simulink model "CK_index_center_main"  (R2023a)
settings: Solver=VariableStepAuto  StartTime=0.0  StopTime=100  RelTol=1e-3
undefined symbols (not defined in the file): a0, a1, a2, a_i_notTop, a_i_Top, Alpha, Alpha1, Alpha2, Alpha3, b0, b1, b2, Cr, d1, d2, DCLV3, DCLV3signal, DCyt, ds, DSstemcells, dw, K1, K2, Kh1, Kh2, n, ra, rclv, rclvs, rcyt, receptor_i1, receptor_i2, receptor_i3, receptor_i4, receptor_i5, receptor_i6, receptor_i7, receptor_i8, rsc, rw, V1, Vh1
settings Model: Creator=mosuk  LastModifiedBy=mosuk

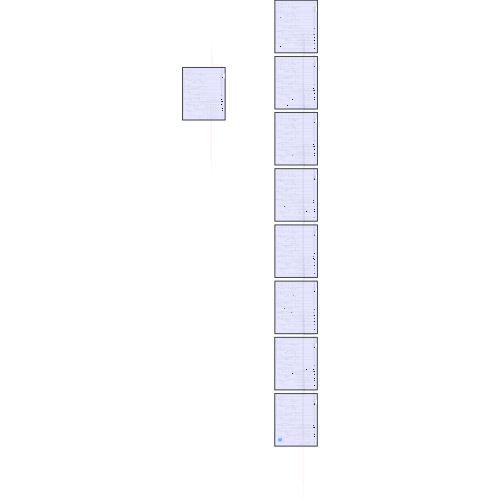
[thumbnail: Simulink's stored preview of the top-level diagram]
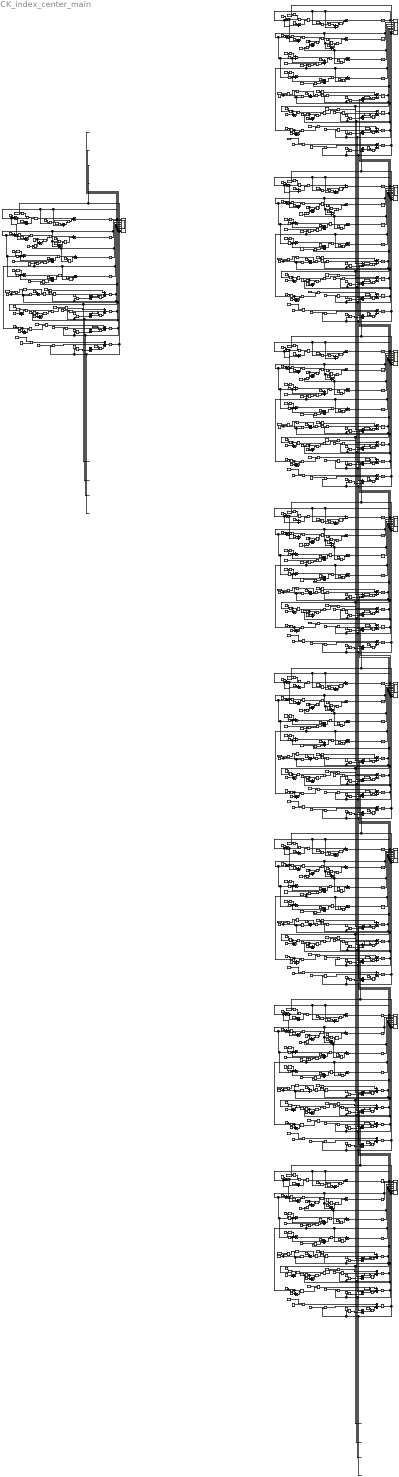
== system CK_index_center_main ==
  note: a_i_notTop
  note: i = 2
  note: i = 3
  note: i = 1
  note: i = 1
  note: i = 4
  note: i = 5
  note: i = 6
  note: i = 7
  note: i = 8
  Constant{100,148,244,292,340,388,436,484,532} (9 alike) : Constant  Value=a1
  Constant{101,149,245,293,341,389,437,485,533} (9 alike) : Constant  Value=ra
  Constant{102,150,246,294,342,390,438,486,534} (9 alike) : Constant  Value=a2
  Constant{103,151,247,295,343,391,439,487,535} (9 alike) : Constant  Value=b1
  Constant{104,152,248,296,344,392,440,488,536} (9 alike) : Constant  Value=n
  Constant{105,109,116,123,125,127,136,153,157,164,171,173,175,184,249,253,260,267,269,271,280,297,301,308,315,317,319,322,324..326,328,345,349,356,363,365,367,376,393,397,404,411,413,415,424,441,445,452,459,461,463,472,489,493,500,507,509,511,520,537,541,548,555,557,559,568} (67 alike) : Constant
  Constant{106,154,250,298,346,394,442,490,538} (9 alike) : Constant  Value=b2
  Constant{107,155,251,299,347,395,443,491,539} (9 alike) : Constant  Value=b0
  Constant{99,108,147,156,243,252,291,300,339,348,387,396,435,444,483,492,531,540} (18 alike) : Constant  Value=10
  Constant{110,158,254,302,350,398,446,494,542} (9 alike) : Constant  Value=d2
  Constant{111,159,255,303,351,399,447,495,543} (9 alike) : Constant  Value=ds
  Constant{112,160,256,304,352,400,448,496,544} (9 alike) : Constant  Value=Alpha1
  Constant{113,161,257,305,353,401,449,497,545} (9 alike) : Constant  Value=rw
  Constant{114,162,258,306,354,402,450,498,546} (9 alike) : Constant  Value=Alpha3
  Constant{115,163,259,307,355,403,451,499,547} (9 alike) : Constant  Value=Cr
  Constant{117,131,165,179,357,371,405,419,453,467,501,515,549,563} (14 alike) : Constant  Value=a_i_notTop
  Constant{118,166,262,310,358,406,454,502,550} (9 alike) : Constant  Value=rclvs
  Constant{119,167,263,311,359,407,455,503,551} (9 alike) : Constant  Value=Kh1
  Constant{120,168,264,312,360,408,456,504,552} (9 alike) : Constant  Value=d1
  Constant{121,169,265,313,361,409,457,505,553} (9 alike) : Constant  Value=Alpha2
  Constant{122,170,266,314,362,410,458,506,554} (9 alike) : Constant  Value=rclv
  Constant{124,172,268,316,364,412,460,508,556} (9 alike) : Constant  Value=rsc
  Constant{126,174,270,318,366,414,462,510,558} (9 alike) : Constant  Value=rcyt
  Constant{128,176,272,320,368,416,464,512,560} (9 alike) : Constant  Value=dw
  Constant{129,177,273,321,369,417,465,513,561} (9 alike) : Constant  Value=Kh2
  Constant{130,132..134,178,180..182,274,276..278,370,372..374,418,420..422,466,468..470,514,516..518,562,564..566} (32 alike) : Constant  Value=2
  Constant{135,183,279,327,375,423,471,519,567} (9 alike) : Constant  Value=Vh1
  Constant{137,185,281,329,377,425,473,521,569} (9 alike) : Constant  Value=DCLV3
  Constant{138,186,282,330,378,426,474,522,570} (9 alike) : Constant  Value=a0
  Constant{139,187,283,331,379,427,475,523,571} (9 alike) : Constant  Value=Alpha
  Constant{140,188,284,332,380,428,476,524,572} (9 alike) : Constant  Value=DCLV3signal
  Constant{141,189,285,333,381,429,477,525,573} (9 alike) : Constant  Value=DCyt
  Constant{142,190,286,334,382,430,478,526,574} (9 alike) : Constant  Value=DSstemcells
  Constant{143,191,287,335,383,431,479,527,575} (9 alike) : Constant  Value=V1
  Constant144 : Constant  Value=receptor_i3
  Constant{97,145,241,289,337,385,433,481,529} (9 alike) : Constant  Value=K1
  Constant{98,146,242,290,338,386,434,482,530} (9 alike) : Constant  Value=K2
  Constant240 : Constant  Value=receptor_i1
  Constant{261,275,309,323} (4 alike) : Constant  Value=a_i_Top
  Constant288 : Constant  Value=receptor_i1
  Constant336 : Constant  Value=receptor_i4
  Constant384 : Constant  Value=receptor_i5
  Constant432 : Constant  Value=receptor_i6
  Constant480 : Constant  Value=receptor_i7
  Constant528 : Constant  Value=receptor_i8
  Constant96 : Constant  Value=receptor_i2
  Divide{22..43,55..131} (99 alike) : Product  Inputs=*/
  Integrator{16..31,40..95} (72 alike) : Integrator
  Math Function{2..3,5..11} (9 alike) : Math  Operator=pow
  Product{72..143,180..431} (324 alike) : Product
  Subtract{68,73..74,76,95,100..101,103,149,154..155,157,176,181..182,184,203,208..209,211,230,235..236,238,257,262..263,265,284,289..290,292,311,316..317,319} (36 alike) : Sum  Inputs=+-+
  Subtract{54,58,65,72,75,80..81,85,92,99,102,107,135,139,146,153,156,161..162,166,173,180,183,188..189,193,200,207,210,215..216,220,227,234,237,242..243,247,254,261,264,269..270,274,281,288,291,296..297,301,308,315,318,323} (54 alike) : Sum  Inputs=+-
  Subtract{55..56,59,61,63..64,67,71,77..79,82..83,86,88,90..91,94,98,104..106,136..137,140,142,144..145,148,152,158..160,163..164,167,169,171..172,175,179,185..187,190..191,194,196,198..199,202,206,212..214,217..218,221,223,225..226,229,233,239..241,244..245,248,250,252..253,256,260,266..268,271..272,275,277,279..280,283,287,293..295,298..299,302,304,306..307,310,314,320..322} (99 alike) : Sum
  Subtract{57,60,84,87,138,141,165,168,192,195,219,222,246,249,273,276,300,303} (18 alike) : Sum  Inputs=+++
  Subtract{62,66,69..70,89,93,96..97,143,147,150..151,170,174,177..178,197,201,204..205,224,228,231..232,251,255,258..259,278,282,285..286,305,309,312..313} (36 alike) : Sum  Inputs=++-
  i -6 : Scope  NumInputPorts=8
  i = {1..8} (8 alike) : Scope  NumInputPorts=8
  wires:
  Constant132/1 -> Product95/1
  Subtract72/1 -> Integrator23/1  "Bp'"
  Constant107/1 -> Subtract59/1
  Constant111/1 -> Product76/2, Product79/1
  Constant139/1 -> Product94/2
  Constant127/1 -> Subtract67/1
  Subtract55/1 -> Divide22/2
  Constant143/1 -> Product99/1
  Subtract76/1 -> Integrator20/1  "Sstemcells'"
  Constant130/1 -> Product93/1
  Constant116/1 -> Subtract61/1
  Product95/1 -> Subtract66/3
  Product87/1 -> Subtract76/2
  Constant133/1 -> Product96/1
  Constant138/1 -> Subtract56/1
  Divide29/1 -> Subtract58/1
  Subtract80/1 -> Integrator16/1  "A'"
  Subtract67/1 -> Divide24/2
  Math Function2/1 -> Product105/2
  Constant122/1 -> Product81/1
  Divide31/1 -> Product85/1
  Product100/1 -> Subtract74/3
  Divide24/1 -> Product89/2
  Constant102/1 -> Product105/1
  Constant120/1 -> Product83/1
  Divide23/1 -> Subtract65/2
  Subtract69/1 -> Product102/2
  Product89/1 -> Subtract76/1
  Divide32/1 -> Product85/2
  Product86/1 -> Subtract64/2, Divide32/1
  Subtract75/1 -> Subtract77/2, Product84/2  "B"
  Subtract70/1 -> Product103/2
  Constant137/1 -> Product101/1
  Product81/1 -> Subtract73/2
  Subtract74/1 -> Integrator18/1  "CLV3signal'"
  Constant118/1 -> Product80/1
  Constant136/1 -> Subtract78/1, Divide26/1
  Constant106/1 -> Product74/1
  Divide22/1 -> Subtract65/1
  Constant98/1 -> Subtract79/1
  Constant114/1 -> Product89/1
  Product73/1 -> Divide23/1
  Constant117/1 -> Product76/1
  Integrator20/1 -> Product86/2, Product79/2, Product78/2, Subtract177/2, i = 2/7, Subtract96/1, Product96/2, Product87/2  "2Sstemcells"
  Product107/1 -> Subtract60/2, Subtract59/2
  Product74/1 -> Subtract60/3
  Product76/1 -> Product78/1
  Product82/1 -> Subtract73/1
  Integrator16/1 -> Product106/2, Product94/1, i = 2/3  "2A"
  Product77/1 -> Subtract74/1
  Divide28/1 -> Subtract80/1
  Constant109/1 -> Subtract60/1
  Subtract79/1 -> Divide27/2
  Constant126/1 -> Product91/1
  Subtract62/1 -> Product101/2
  Product99/1 -> Divide27/1
  Subtract57/1 -> Divide28/2
  Constant115/1 -> Product90/2
  Constant108/1 -> Subtract54/1
  Divide30/1 -> Product77/2
  Integrator21/1 -> Product92/1, Subtract178/2, i = 2/8, Subtract97/1, Product97/2, Product91/2  "2Cyt"
  Constant124/1 -> Product87/1
  Integrator19/1 -> Subtract89/1, Product81/2, Product93/2, Product74/2, Subtract170/2, i = 2/6  "2CLV3"
  Constant101/1 -> Product106/1
  Divide26/1 -> Product98/2
  Subtract61/1 -> Divide30/2
  Constant112/1 -> Product77/1
  Product105/1 -> Subtract57/3
  Product96/1 -> Subtract69/3
  Subtract77/1 -> Divide25/2
  Constant100/1 -> Product104/1
  Constant104/1 -> Math Function2/2
  Integrator18/1 -> Product95/2, Product80/2, Subtract93/1, Product83/2, Subtract174/2, i = 2/5  "2CLV3signal"
  Subtract78/1 -> Divide26/2
  Subtract65/1 -> Integrator22/1  "AHPTp'"
  Subtract71/1 -> Divide23/2
  Product72/1 -> Divide22/1
  Integrator22/1 -> Subtract71/2, Product73/2, Product84/1, Subtract54/2, i = 2/1  "2AHPTp"
  Product79/1 -> Subtract61/2
  Constant119/1 -> Subtract55/1
  Constant110/1 -> Product86/1
  Constant103/1 -> Product107/1
  Subtract56/1 -> Divide28/1
  Subtract64/1 -> Divide32/2
  Integrator23/1 -> Subtract79/2, Product99/2, Subtract75/2, Product107/2, Product104/2, i = 2/2  "2Bp"
  Product90/1 -> Subtract68/1
  Subtract66/1 -> Product100/2
  Subtract58/1 -> Integrator17/1  "WUS'"
  Product91/1 -> Subtract68/2
  Integrator17/1 -> Product75/2, Product88/2, Math Function2/1, i = 2/4  "2WUS"
  Constant105/1 -> Subtract57/1
  Product106/1 -> Subtract80/2
  Constant121/1 -> Product82/1
  Product85/1 -> Product82/2
  Constant125/1 -> Subtract63/1
  Product94/1 -> Subtract78/2
  Product93/1 -> Subtract62/3
  Product83/1 -> Divide31/1, Subtract63/2
  Product101/1 -> Subtract73/3
  Constant134/1 -> Product97/1
  Divide25/1 -> Product98/1
  Product97/1 -> Subtract70/3
  Constant99/1 -> Subtract75/1
  Subtract63/1 -> Divide31/2
  Product75/1 -> Subtract58/2
  Constant128/1 -> Product88/1
  Constant123/1 -> Subtract64/1
  Constant96/1 -> Product92/2
  Product78/1 -> Divide30/1
  Product84/1 -> Divide25/1
  Product104/1 -> Subtract57/2, Subtract56/2
  Constant113/1 -> Product75/1
  Product92/1 -> Product72/1
  Constant129/1 -> Subtract71/1
  Constant131/1 -> Product90/1
  Divide27/1 -> Subtract72/2
  Constant97/1 -> Subtract77/1
  Subtract73/1 -> Integrator19/1  "CLV3'"
  Constant140/1 -> Product100/1
  Subtract59/1 -> Divide29/1
  Subtract60/1 -> Divide29/2
  Constant135/1 -> Product73/1
  Constant142/1 -> Product102/1
  Product103/1 -> Subtract68/3
  Subtract68/1 -> Integrator21/1  "Cyt'"
  Constant141/1 -> Product103/1
  Subtract54/1 -> Subtract55/2, Product72/2  "AHPT"
  Product102/1 -> Subtract76/3
  Product88/1 -> Subtract67/2, Divide24/1
  Product98/1 -> Subtract72/1
  Product80/1 -> Subtract74/2
  Constant180/1 -> Product131/1
  Subtract99/1 -> Integrator31/1  "Bp'"
  Constant155/1 -> Subtract86/1
  Constant159/1 -> Product112/2, Product115/1
  Constant187/1 -> Product130/2
  Constant175/1 -> Subtract94/1
  Subtract82/1 -> Divide33/2
  Constant191/1 -> Product135/1
  Subtract103/1 -> Integrator28/1  "Sstemcells'"
  Constant178/1 -> Product129/1
  Constant164/1 -> Subtract88/1
  Product131/1 -> Subtract93/3
  Product123/1 -> Subtract103/2
  Constant181/1 -> Product132/1
  Constant186/1 -> Subtract83/1
  Divide40/1 -> Subtract85/1
  Subtract107/1 -> Integrator24/1  "A'"
  Subtract94/1 -> Divide35/2
  Math Function3/1 -> Product141/2
  Constant170/1 -> Product117/1
  Divide42/1 -> Product121/1
  Product136/1 -> Subtract101/3
  Divide35/1 -> Product125/2
  Constant150/1 -> Product141/1
  Constant168/1 -> Product119/1
  Divide34/1 -> Subtract92/2
  Subtract96/1 -> Product138/2
  Product125/1 -> Subtract103/1
  Divide43/1 -> Product121/2
  Product122/1 -> Subtract91/2, Divide43/1
  Subtract102/1 -> Subtract104/2, Product120/2  "B"
  Subtract97/1 -> Product139/2
  Constant185/1 -> Product137/1
  Product117/1 -> Subtract100/2
  Subtract101/1 -> Integrator26/1  "CLV3signal'"
  Constant166/1 -> Product116/1
  Constant184/1 -> Subtract105/1, Divide37/1
  Constant154/1 -> Product110/1
  Divide33/1 -> Subtract92/1
  Constant146/1 -> Subtract106/1
  Constant162/1 -> Product125/1
  Product109/1 -> Divide34/1
  Constant165/1 -> Product112/1
  Integrator28/1 -> Product122/2, Product115/2, Product114/2, Subtract69/2, i = 3/7, Subtract204/1, Product132/2, Product123/2  "3Sstemcells"
  Product143/1 -> Subtract87/2, Subtract86/2
  Product110/1 -> Subtract87/3
  Product112/1 -> Product114/1
  Product118/1 -> Subtract100/1
  Integrator24/1 -> Product142/2, Product130/1, i = 3/3  "3A"
  Product113/1 -> Subtract101/1
  Divide39/1 -> Subtract107/1
  Constant157/1 -> Subtract87/1
  Subtract106/1 -> Divide38/2
  Constant174/1 -> Product127/1
  Subtract89/1 -> Product137/2
  Product135/1 -> Divide38/1
  Subtract84/1 -> Divide39/2
  Constant163/1 -> Product126/2
  Constant156/1 -> Subtract81/1
  Divide41/1 -> Product113/2
  Integrator29/1 -> Subtract70/2, Product128/1, i = 3/8, Subtract205/1, Product133/2, Product127/2  "3Cyt"
  Constant172/1 -> Product123/1
  Integrator27/1 -> Subtract197/1, Product117/2, Product129/2, Product110/2, Subtract62/2, i = 3/6  "3CLV3"
  Constant149/1 -> Product142/1
  Divide37/1 -> Product134/2
  Subtract88/1 -> Divide41/2
  Constant160/1 -> Product113/1
  Product141/1 -> Subtract84/3
  Product132/1 -> Subtract96/3
  Subtract104/1 -> Divide36/2
  Constant148/1 -> Product140/1
  Constant152/1 -> Math Function3/2
  Integrator26/1 -> Product131/2, Product116/2, Subtract201/1, Product119/2, Subtract66/2, i = 3/5  "3CLV3signal"
  Subtract105/1 -> Divide37/2
  Subtract92/1 -> Integrator30/1  "AHPTp'"
  Subtract98/1 -> Divide34/2
  Product108/1 -> Divide33/1
  Integrator30/1 -> Subtract98/2, Product109/2, Product120/1, Subtract81/2, i = 3/1  "3AHPTp"
  Product115/1 -> Subtract88/2
  Constant167/1 -> Subtract82/1
  Constant158/1 -> Product122/1
  Constant151/1 -> Product143/1
  Subtract83/1 -> Divide39/1
  Subtract91/1 -> Divide43/2
  Integrator31/1 -> Subtract106/2, Product135/2, Subtract102/2, Product143/2, Product140/2, i = 3/2  "3Bp"
  Product126/1 -> Subtract95/1
  Subtract93/1 -> Product136/2
  Subtract85/1 -> Integrator25/1  "WUS'"
  Product127/1 -> Subtract95/2
  Integrator25/1 -> Product111/2, Product124/2, Math Function3/1, i = 3/4  "3WUS"
  Constant153/1 -> Subtract84/1
  Product142/1 -> Subtract107/2
  Constant169/1 -> Product118/1
  Product121/1 -> Product118/2
  Constant173/1 -> Subtract90/1
  Product130/1 -> Subtract105/2
  Product129/1 -> Subtract89/3
  Product119/1 -> Divide42/1, Subtract90/2
  Product137/1 -> Subtract100/3
  Constant182/1 -> Product133/1
  Divide36/1 -> Product134/1
  Product133/1 -> Subtract97/3
  Constant147/1 -> Subtract102/1
  Subtract90/1 -> Divide42/2
  Product111/1 -> Subtract85/2
  Constant176/1 -> Product124/1
  Constant171/1 -> Subtract91/1
  Constant144/1 -> Product128/2
  Product114/1 -> Divide41/1
  Product120/1 -> Divide36/1
  Product140/1 -> Subtract84/2, Subtract83/2
  Constant161/1 -> Product111/1
  Product128/1 -> Product108/1
  Constant177/1 -> Subtract98/1
  Constant179/1 -> Product126/1
  Divide38/1 -> Subtract99/2
  Constant145/1 -> Subtract104/1
  Subtract100/1 -> Integrator27/1  "CLV3'"
  Constant188/1 -> Product136/1
  Subtract86/1 -> Divide40/1
  Subtract87/1 -> Divide40/2
  Constant183/1 -> Product109/1
  Constant190/1 -> Product138/1
  Product139/1 -> Subtract95/3
  Subtract95/1 -> Integrator29/1  "Cyt'"
  Constant189/1 -> Product139/1
  Subtract81/1 -> Subtract82/2, Product108/2  "AHPT"
  Product138/1 -> Subtract103/3
  Product124/1 -> Subtract94/2, Divide35/1
  Product134/1 -> Subtract99/1
  Product116/1 -> Subtract101/2
  Constant276/1 -> Product203/1
  Subtract153/1 -> Integrator47/1  "Bp'"
  Constant251/1 -> Subtract140/1
  Constant255/1 -> Product184/2, Product187/1
  Constant283/1 -> Product202/2
  Constant271/1 -> Subtract148/1
  Subtract136/1 -> Divide55/2
  Constant287/1 -> Product207/1
  Subtract157/1 -> Integrator44/1  "Sstemcells'"
  Constant274/1 -> Product201/1
  Constant260/1 -> Subtract142/1
  Product203/1 -> Subtract147/3
  Product195/1 -> Subtract157/2
  Constant277/1 -> Product204/1
  Constant282/1 -> Subtract137/1
  Divide62/1 -> Subtract139/1
  Subtract161/1 -> Integrator40/1  "A'"
  Subtract148/1 -> Divide57/2
  Math Function5/1 -> Product213/2
  Constant266/1 -> Product189/1
  Divide64/1 -> Product193/1
  Product208/1 -> Subtract155/3
  Divide57/1 -> Product197/2
  Constant246/1 -> Product213/1
  Constant264/1 -> Product191/1
  Divide56/1 -> Subtract146/2
  Subtract150/1 -> Product210/2
  Product197/1 -> Subtract157/1
  Divide65/1 -> Product193/2
  Product194/1 -> Subtract145/2, Divide65/1
  Subtract156/1 -> Subtract158/2, Product192/2  "B"
  Subtract151/1 -> Product211/2
  Constant281/1 -> Product209/1
  Product189/1 -> Subtract154/2
  Subtract155/1 -> Integrator42/1  "CLV3signal'"
  Constant262/1 -> Product188/1
  Constant280/1 -> Subtract159/1, Divide59/1
  Constant250/1 -> Product182/1
  Divide55/1 -> Subtract146/1
  Constant242/1 -> Subtract160/1
  Constant258/1 -> Product197/1
  Product181/1 -> Divide56/1
  Constant261/1 -> Product184/1
  Integrator44/1 -> Product194/2, Product187/2, Product186/2, i -6/7, Product204/2, Product195/2  "0Sstemcells"
  Product215/1 -> Subtract141/2, Subtract140/2
  Product182/1 -> Subtract141/3
  Product184/1 -> Product186/1
  Product190/1 -> Subtract154/1
  Integrator40/1 -> Product214/2, Product202/1, i -6/3  "2A"
  Product185/1 -> Subtract155/1
  Divide61/1 -> Subtract161/1
  Constant253/1 -> Subtract141/1
  Subtract160/1 -> Divide60/2
  Constant270/1 -> Product199/1
  Subtract143/1 -> Product209/2
  Product207/1 -> Divide60/1
  Subtract138/1 -> Divide61/2
  Constant259/1 -> Product198/2
  Constant252/1 -> Subtract135/1
  Divide63/1 -> Product185/2
  Integrator45/1 -> Product200/1, i -6/8, Product205/2, Product199/2  "0Cyt"
  Constant268/1 -> Product195/1
  Integrator43/1 -> Product189/2, Product201/2, Product182/2, i -6/6  "0CLV3"
  Constant245/1 -> Product214/1
  Divide59/1 -> Product206/2
  Subtract142/1 -> Divide63/2
  Constant256/1 -> Product185/1
  Product213/1 -> Subtract138/3
  Product204/1 -> Subtract150/3
  Subtract158/1 -> Divide58/2
  Constant244/1 -> Product212/1
  Constant248/1 -> Math Function5/2
  Integrator42/1 -> Product203/2, Product188/2, Product191/2, i -6/5  "0CLV3signal"
  Subtract159/1 -> Divide59/2
  Subtract146/1 -> Integrator46/1  "AHPTp'"
  Subtract152/1 -> Divide56/2
  Product180/1 -> Divide55/1
  Integrator46/1 -> Subtract152/2, Product181/2, Product192/1, Subtract135/2, i -6/1  "2AHPTp"
  Product187/1 -> Subtract142/2
  Constant263/1 -> Subtract136/1
  Constant254/1 -> Product194/1
  Constant247/1 -> Product215/1
  Subtract137/1 -> Divide61/1
  Subtract145/1 -> Divide65/2
  Integrator47/1 -> Subtract160/2, Product207/2, Subtract156/2, Product215/2, Product212/2, i -6/2  "2Bp"
  Product198/1 -> Subtract149/1
  Subtract147/1 -> Product208/2
  Subtract139/1 -> Integrator41/1  "WUS'"
  Product199/1 -> Subtract149/2
  Integrator41/1 -> Product183/2, Product196/2, Math Function5/1, i -6/4  "0WUS"
  Constant249/1 -> Subtract138/1
  Product214/1 -> Subtract161/2
  Constant265/1 -> Product190/1
  Product193/1 -> Product190/2
  Constant269/1 -> Subtract144/1
  Product202/1 -> Subtract159/2
  Product201/1 -> Subtract143/3
  Product191/1 -> Divide64/1, Subtract144/2
  Product209/1 -> Subtract154/3
  Constant278/1 -> Product205/1
  Divide58/1 -> Product206/1
  Product205/1 -> Subtract151/3
  Constant243/1 -> Subtract156/1
  Subtract144/1 -> Divide64/2
  Product183/1 -> Subtract139/2
  Constant272/1 -> Product196/1
  Constant267/1 -> Subtract145/1
  Constant240/1 -> Product200/2
  Product186/1 -> Divide63/1
  Product192/1 -> Divide58/1
  Product212/1 -> Subtract138/2, Subtract137/2
  Constant257/1 -> Product183/1
  Product200/1 -> Product180/1
  Constant273/1 -> Subtract152/1
  Constant275/1 -> Product198/1
  Divide60/1 -> Subtract153/2
  Constant241/1 -> Subtract158/1
  Subtract154/1 -> Integrator43/1  "CLV3'"
  Constant284/1 -> Product208/1
  Subtract140/1 -> Divide62/1
  Subtract141/1 -> Divide62/2
  Constant279/1 -> Product181/1
  Constant286/1 -> Product210/1
  Product211/1 -> Subtract149/3
  Subtract149/1 -> Integrator45/1  "Cyt'"
  Constant285/1 -> Product211/1
  Subtract135/1 -> Subtract136/2, Product180/2  "AHPT"
  Product210/1 -> Subtract157/3
  Product196/1 -> Subtract148/2, Divide57/1
  Product206/1 -> Subtract153/1
  Product188/1 -> Subtract155/2
  Constant324/1 -> Product239/1
  Subtract180/1 -> Integrator55/1  "Bp'"
  Constant299/1 -> Subtract167/1
  Constant303/1 -> Product220/2, Product223/1
  Constant331/1 -> Product238/2
  Constant319/1 -> Subtract175/1
  Subtract163/1 -> Divide66/2
  Constant335/1 -> Product243/1
  Subtract184/1 -> Integrator52/1  "Sstemcells'"
  Constant322/1 -> Product237/1
  Constant308/1 -> Subtract169/1
  Product239/1 -> Subtract174/3
  Product231/1 -> Subtract184/2
  Constant325/1 -> Product240/1
  Constant330/1 -> Subtract164/1
  Divide73/1 -> Subtract166/1
  Subtract188/1 -> Integrator48/1  "A'"
  Subtract175/1 -> Divide68/2
  Math Function6/1 -> Product249/2
  Constant314/1 -> Product225/1
  Divide75/1 -> Product229/1
  Product244/1 -> Subtract182/3
  Divide68/1 -> Product233/2
  Constant294/1 -> Product249/1
  Constant312/1 -> Product227/1
  Divide67/1 -> Subtract173/2
  Subtract177/1 -> Product246/2
  Product233/1 -> Subtract184/1
  Divide76/1 -> Product229/2
  Product230/1 -> Subtract172/2, Divide76/1
  Subtract183/1 -> Subtract185/2, Product228/2  "B"
  Subtract178/1 -> Product247/2
  Constant329/1 -> Product245/1
  Product225/1 -> Subtract181/2
  Subtract182/1 -> Integrator50/1  "CLV3signal'"
  Constant310/1 -> Product224/1
  Constant328/1 -> Subtract186/1, Divide70/1
  Constant298/1 -> Product218/1
  Divide66/1 -> Subtract173/1
  Constant290/1 -> Subtract187/1
  Constant306/1 -> Product233/1
  Product217/1 -> Divide67/1
  Constant309/1 -> Product220/1
  Integrator52/1 -> Product230/2, Product223/2, Product222/2, i = 1/7, Subtract69/1, Product240/2, Product231/2  "1Sstemcells"
  Product251/1 -> Subtract168/2, Subtract167/2
  Product218/1 -> Subtract168/3
  Product220/1 -> Product222/1
  Product226/1 -> Subtract181/1
  Integrator48/1 -> Product250/2, Product238/1, i = 1/3  "1A"
  Product221/1 -> Subtract182/1
  Divide72/1 -> Subtract188/1
  Constant301/1 -> Subtract168/1
  Subtract187/1 -> Divide71/2
  Constant318/1 -> Product235/1
  Subtract170/1 -> Product245/2
  Product243/1 -> Divide71/1
  Subtract165/1 -> Divide72/2
  Constant307/1 -> Product234/2
  Constant300/1 -> Subtract162/1
  Divide74/1 -> Product221/2
  Integrator53/1 -> Product236/1, i = 1/8, Subtract70/1, Product241/2, Product235/2  "1Cyt"
  Constant316/1 -> Product231/1
  Integrator51/1 -> Subtract62/1, Product225/2, Product237/2, Product218/2, i = 1/6  "1CLV3"
  Constant293/1 -> Product250/1
  Divide70/1 -> Product242/2
  Subtract169/1 -> Divide74/2
  Constant304/1 -> Product221/1
  Product249/1 -> Subtract165/3
  Product240/1 -> Subtract177/3
  Subtract185/1 -> Divide69/2
  Constant292/1 -> Product248/1
  Constant296/1 -> Math Function6/2
  Integrator50/1 -> Product239/2, Product224/2, Subtract66/1, Product227/2, i = 1/5  "1CLV3signal"
  Subtract186/1 -> Divide70/2
  Subtract173/1 -> Integrator54/1  "AHPTp'"
  Subtract179/1 -> Divide67/2
  Product216/1 -> Divide66/1
  Integrator54/1 -> Subtract179/2, Product217/2, Product228/1, Subtract162/2, i = 1/1  "1AHPTp"
  Product223/1 -> Subtract169/2
  Constant311/1 -> Subtract163/1
  Constant302/1 -> Product230/1
  Constant295/1 -> Product251/1
  Subtract164/1 -> Divide72/1
  Subtract172/1 -> Divide76/2
  Integrator55/1 -> Subtract187/2, Product243/2, Subtract183/2, Product251/2, Product248/2, i = 1/2  "1Bp"
  Product234/1 -> Subtract176/1
  Subtract174/1 -> Product244/2
  Subtract166/1 -> Integrator49/1  "WUS'"
  Product235/1 -> Subtract176/2
  Integrator49/1 -> Product219/2, Product232/2, Math Function6/1, i = 1/4  "1WUS"
  Constant297/1 -> Subtract165/1
  Product250/1 -> Subtract188/2
  Constant313/1 -> Product226/1
  Product229/1 -> Product226/2
  Constant317/1 -> Subtract171/1
  Product238/1 -> Subtract186/2
  Product237/1 -> Subtract170/3
  Product227/1 -> Divide75/1, Subtract171/2
  Product245/1 -> Subtract181/3
  Constant326/1 -> Product241/1
  Divide69/1 -> Product242/1
  Product241/1 -> Subtract178/3
  Constant291/1 -> Subtract183/1
  Subtract171/1 -> Divide75/2
  Product219/1 -> Subtract166/2
  Constant320/1 -> Product232/1
  Constant315/1 -> Subtract172/1
  Constant288/1 -> Product236/2
  Product222/1 -> Divide74/1
  Product228/1 -> Divide69/1
  Product248/1 -> Subtract165/2, Subtract164/2
  Constant305/1 -> Product219/1
  Product236/1 -> Product216/1
  Constant321/1 -> Subtract179/1
  Constant323/1 -> Product234/1
  Divide71/1 -> Subtract180/2
  Constant289/1 -> Subtract185/1
  Subtract181/1 -> Integrator51/1  "CLV3'"
  Constant332/1 -> Product244/1
  Subtract167/1 -> Divide73/1
  Subtract168/1 -> Divide73/2
  Constant327/1 -> Product217/1
  Constant334/1 -> Product246/1
  Product247/1 -> Subtract176/3
  Subtract176/1 -> Integrator53/1  "Cyt'"
  Constant333/1 -> Product247/1
  Subtract162/1 -> Subtract163/2, Product216/2  "AHPT"
  Product246/1 -> Subtract184/3
  Product232/1 -> Subtract175/2, Divide68/1
  Product242/1 -> Subtract180/1
  Product224/1 -> Subtract182/2
  Subtract210/1 -> Subtract212/2, Product264/2  "B"
  Product256/1 -> Product258/1
  Divide78/1 -> Subtract200/2
  Product281/1 -> Subtract208/3
  Product273/1 -> Subtract197/3
  Divide81/1 -> Product278/2
  Subtract193/1 -> Integrator57/1  "WUS'"
  Integrator56/1 -> Product286/2, Product274/1, i = 4/3  "4A"
  Constant360/1 -> Product263/1
  Subtract189/1 -> Subtract190/2, Product252/2  "AHPT"
  Integrator63/1 -> Subtract214/2, Product279/2, Subtract210/2, Product287/2, Product284/2, i = 4/2  "4Bp"
  Constant338/1 -> Subtract214/1
  Product282/1 -> Subtract211/3
  Math Function7/1 -> Product285/2
  Product283/1 -> Subtract203/3
  Subtract200/1 -> Integrator62/1  "AHPTp'"
  Product284/1 -> Subtract192/2, Subtract191/2
  Product261/1 -> Subtract208/2
  Constant380/1 -> Product280/1
  Constant336/1 -> Product272/2
  Constant381/1 -> Product283/1
  Product266/1 -> Subtract199/2, Divide87/1
  Product274/1 -> Subtract213/2
  Constant374/1 -> Product277/1
  Subtract212/1 -> Divide80/2
  Constant355/1 -> Product270/2
  Subtract197/1 -> Product281/2
  Constant378/1 -> Subtract191/1
  Product270/1 -> Subtract203/1
  Product267/1 -> Subtract211/2
  Constant371/1 -> Product270/1
  Constant345/1 -> Subtract192/1
  Constant375/1 -> Product253/1
  Divide79/1 -> Product269/2
  Subtract215/1 -> Integrator56/1  "A'"
  Constant363/1 -> Subtract199/1
  Constant372/1 -> Product275/1
  Constant344/1 -> Math Function7/2
  Subtract211/1 -> Integrator60/1  "Sstemcells'"
  Product268/1 -> Subtract202/2, Divide79/1
  Constant353/1 -> Product255/1
  Constant359/1 -> Subtract190/1
  Constant346/1 -> Product254/1
  Subtract203/1 -> Integrator61/1  "Cyt'"
  Product278/1 -> Subtract207/1
  Subtract194/1 -> Divide84/1
  Divide80/1 -> Product278/1
  Product258/1 -> Divide85/1
  Product272/1 -> Product252/1
  Subtract196/1 -> Divide85/2
  Subtract195/1 -> Divide84/2
  Constant369/1 -> Subtract206/1
  Constant354/1 -> Product269/1
  Divide82/1 -> Subtract207/2
  Subtract208/1 -> Integrator59/1  "CLV3'"
  Constant382/1 -> Product282/1
  Constant337/1 -> Subtract212/1
  Constant358/1 -> Product260/1
  Product277/1 -> Subtract205/3
  Product254/1 -> Subtract195/3
  Product255/1 -> Subtract193/2
  Constant368/1 -> Product268/1
  Product276/1 -> Subtract204/3
  Subtract198/1 -> Divide86/2
  Product260/1 -> Subtract209/2
  Constant365/1 -> Subtract198/1
  Product263/1 -> Divide86/1, Subtract198/2
  Product286/1 -> Subtract215/2
  Product265/1 -> Product262/2
  Constant343/1 -> Product287/1
  Constant357/1 -> Product256/1
  Subtract204/1 -> Product282/2
  Subtract201/1 -> Product280/2
  Integrator57/1 -> Product255/2, Product268/2, Math Function7/1, i = 4/4  "4WUS"
  Constant349/1 -> Subtract195/1
  Constant361/1 -> Product262/1
  Product271/1 -> Subtract203/2
  Constant376/1 -> Subtract213/1, Divide81/1
  Subtract199/1 -> Divide87/2
  Constant350/1 -> Product266/1
  Subtract191/1 -> Divide83/1
  Integrator58/1 -> Product275/2, Product260/2, Subtract228/1, Product263/2, Subtract93/2, i = 4/5  "4CLV3signal"
  Constant339/1 -> Subtract210/1
  Product259/1 -> Subtract196/2
  Subtract190/1 -> Divide77/2
  Integrator62/1 -> Subtract206/2, Product253/2, Product264/1, Subtract189/2, i = 4/1  "4AHPTp"
  Subtract213/1 -> Divide81/2
  Constant340/1 -> Product284/1
  Constant352/1 -> Product257/1
  Constant341/1 -> Product286/1
  Constant367/1 -> Subtract202/1
  Product262/1 -> Subtract208/1
  Subtract206/1 -> Divide78/2
  Integrator59/1 -> Subtract224/1, Product261/2, Product273/2, Product254/2, Subtract89/2, i = 4/6  "4CLV3"
  Constant366/1 -> Product271/1
  Product252/1 -> Divide77/1
  Constant379/1 -> Product274/2
  Constant364/1 -> Product267/1
  Divide85/1 -> Product257/2
  Constant348/1 -> Subtract189/1
  Subtract192/1 -> Divide83/2
  Product279/1 -> Divide82/1
  Divide83/1 -> Subtract215/1
  Subtract214/1 -> Divide82/2
  Product257/1 -> Subtract209/1
  Product269/1 -> Subtract211/1
  Divide77/1 -> Subtract200/1
  Product285/1 -> Subtract192/3
  Subtract209/1 -> Integrator58/1  "CLV3signal'"
  Product253/1 -> Divide78/1
  Product287/1 -> Subtract195/2, Subtract194/2
  Integrator61/1 -> Subtract97/2, Product272/1, i = 4/8, Subtract232/1, Product277/2, Product271/2  "4Cyt"
  Integrator60/1 -> Product266/2, Product259/2, Product258/2, Subtract96/2, i = 4/7, Subtract231/1, Product276/2, Product267/2  "4Sstemcells"
  Subtract205/1 -> Product283/2
  Constant342/1 -> Product285/1
  Constant377/1 -> Product281/1
  Divide86/1 -> Product265/1
  Product280/1 -> Subtract209/3
  Divide87/1 -> Product265/2
  Subtract202/1 -> Divide79/2
  Divide84/1 -> Subtract193/1
  Constant373/1 -> Product276/1
  Constant362/1 -> Product261/1
  Product264/1 -> Divide80/1
  Constant370/1 -> Product273/1
  Constant383/1 -> Product279/1
  Constant347/1 -> Subtract194/1
  Constant356/1 -> Subtract196/1
  Constant351/1 -> Product256/2, Product259/1
  Product275/1 -> Subtract201/3
  Subtract207/1 -> Integrator63/1  "Bp'"
  Subtract237/1 -> Subtract239/2, Product300/2  "B"
  Product292/1 -> Product294/1
  Divide89/1 -> Subtract227/2
  Product317/1 -> Subtract235/3
  Product309/1 -> Subtract224/3
  Divide92/1 -> Product314/2
  Subtract220/1 -> Integrator65/1  "WUS'"
  Integrator64/1 -> Product322/2, Product310/1, i = 5/3  "5A"
  Constant408/1 -> Product299/1
  Subtract216/1 -> Subtract217/2, Product288/2  "AHPT"
  Integrator71/1 -> Subtract241/2, Product315/2, Subtract237/2, Product323/2, Product320/2, i = 5/2  "5Bp"
  Constant386/1 -> Subtract241/1
  Product318/1 -> Subtract238/3
  Math Function8/1 -> Product321/2
  Product319/1 -> Subtract230/3
  Subtract227/1 -> Integrator70/1  "AHPTp'"
  Product320/1 -> Subtract219/2, Subtract218/2
  Product297/1 -> Subtract235/2
  Constant428/1 -> Product316/1
  Constant384/1 -> Product308/2
  Constant429/1 -> Product319/1
  Product302/1 -> Subtract226/2, Divide98/1
  Product310/1 -> Subtract240/2
  Constant422/1 -> Product313/1
  Subtract239/1 -> Divide91/2
  Constant403/1 -> Product306/2
  Subtract224/1 -> Product317/2
  Constant426/1 -> Subtract218/1
  Product306/1 -> Subtract230/1
  Product303/1 -> Subtract238/2
  Constant419/1 -> Product306/1
  Constant393/1 -> Subtract219/1
  Constant423/1 -> Product289/1
  Divide90/1 -> Product305/2
  Subtract242/1 -> Integrator64/1  "A'"
  Constant411/1 -> Subtract226/1
  Constant420/1 -> Product311/1
  Constant392/1 -> Math Function8/2
  Subtract238/1 -> Integrator68/1  "Sstemcells'"
  Product304/1 -> Subtract229/2, Divide90/1
  Constant401/1 -> Product291/1
  Constant407/1 -> Subtract217/1
  Constant394/1 -> Product290/1
  Subtract230/1 -> Integrator69/1  "Cyt'"
  Product314/1 -> Subtract234/1
  Subtract221/1 -> Divide95/1
  Divide91/1 -> Product314/1
  Product294/1 -> Divide96/1
  Product308/1 -> Product288/1
  Subtract223/1 -> Divide96/2
  Subtract222/1 -> Divide95/2
  Constant417/1 -> Subtract233/1
  Constant402/1 -> Product305/1
  Divide93/1 -> Subtract234/2
  Subtract235/1 -> Integrator67/1  "CLV3'"
  Constant430/1 -> Product318/1
  Constant385/1 -> Subtract239/1
  Constant406/1 -> Product296/1
  Product313/1 -> Subtract232/3
  Product290/1 -> Subtract222/3
  Product291/1 -> Subtract220/2
  Constant416/1 -> Product304/1
  Product312/1 -> Subtract231/3
  Subtract225/1 -> Divide97/2
  Product296/1 -> Subtract236/2
  Constant413/1 -> Subtract225/1
  Product299/1 -> Divide97/1, Subtract225/2
  Product322/1 -> Subtract242/2
  Product301/1 -> Product298/2
  Constant391/1 -> Product323/1
  Constant405/1 -> Product292/1
  Subtract231/1 -> Product318/2
  Subtract228/1 -> Product316/2
  Integrator65/1 -> Product291/2, Product304/2, Math Function8/1, i = 5/4  "5WUS"
  Constant397/1 -> Subtract222/1
  Constant409/1 -> Product298/1
  Product307/1 -> Subtract230/2
  Constant424/1 -> Subtract240/1, Divide92/1
  Subtract226/1 -> Divide98/2
  Constant398/1 -> Product302/1
  Subtract218/1 -> Divide94/1
  Integrator66/1 -> Product311/2, Product296/2, Subtract255/1, Product299/2, Subtract201/2, i = 5/5  "5CLV3signal"
  Constant387/1 -> Subtract237/1
  Product295/1 -> Subtract223/2
  Subtract217/1 -> Divide88/2
  Integrator70/1 -> Subtract233/2, Product289/2, Product300/1, Subtract216/2, i = 5/1  "5AHPTp"
  Subtract240/1 -> Divide92/2
  Constant388/1 -> Product320/1
  Constant400/1 -> Product293/1
  Constant389/1 -> Product322/1
  Constant415/1 -> Subtract229/1
  Product298/1 -> Subtract235/1
  Subtract233/1 -> Divide89/2
  Integrator67/1 -> Subtract251/1, Product297/2, Product309/2, Product290/2, Subtract197/2, i = 5/6  "5CLV3"
  Constant414/1 -> Product307/1
  Product288/1 -> Divide88/1
  Constant427/1 -> Product310/2
  Constant412/1 -> Product303/1
  Divide96/1 -> Product293/2
  Constant396/1 -> Subtract216/1
  Subtract219/1 -> Divide94/2
  Product315/1 -> Divide93/1
  Divide94/1 -> Subtract242/1
  Subtract241/1 -> Divide93/2
  Product293/1 -> Subtract236/1
  Product305/1 -> Subtract238/1
  Divide88/1 -> Subtract227/1
  Product321/1 -> Subtract219/3
  Subtract236/1 -> Integrator66/1  "CLV3signal'"
  Product289/1 -> Divide89/1
  Product323/1 -> Subtract222/2, Subtract221/2
  Integrator69/1 -> Subtract205/2, Product308/1, i = 5/8, Subtract259/1, Product313/2, Product307/2  "5Cyt"
  Integrator68/1 -> Product302/2, Product295/2, Product294/2, Subtract204/2, i = 5/7, Subtract258/1, Product312/2, Product303/2  "5Sstemcells"
  Subtract232/1 -> Product319/2
  Constant390/1 -> Product321/1
  Constant425/1 -> Product317/1
  Divide97/1 -> Product301/1
  Product316/1 -> Subtract236/3
  Divide98/1 -> Product301/2
  Subtract229/1 -> Divide90/2
  Divide95/1 -> Subtract220/1
  Constant421/1 -> Product312/1
  Constant410/1 -> Product297/1
  Product300/1 -> Divide91/1
  Constant418/1 -> Product309/1
  Constant431/1 -> Product315/1
  Constant395/1 -> Subtract221/1
  Constant404/1 -> Subtract223/1
  Constant399/1 -> Product292/2, Product295/1
  Product311/1 -> Subtract228/3
  Subtract234/1 -> Integrator71/1  "Bp'"
  Subtract264/1 -> Subtract266/2, Product336/2  "B"
  Product328/1 -> Product330/1
  Divide100/1 -> Subtract254/2
  Product353/1 -> Subtract262/3
  Product345/1 -> Subtract251/3
  Divide103/1 -> Product350/2
  Subtract247/1 -> Integrator73/1  "WUS'"
  Integrator72/1 -> Product358/2, Product346/1, i = 6/3  "6A"
  Constant456/1 -> Product335/1
  Subtract243/1 -> Subtract244/2, Product324/2  "AHPT"
  Integrator79/1 -> Subtract268/2, Product351/2, Subtract264/2, Product359/2, Product356/2, i = 6/2  "6Bp"
  Constant434/1 -> Subtract268/1
  Product354/1 -> Subtract265/3
  Math Function9/1 -> Product357/2
  Product355/1 -> Subtract257/3
  Subtract254/1 -> Integrator78/1  "AHPTp'"
  Product356/1 -> Subtract246/2, Subtract245/2
  Product333/1 -> Subtract262/2
  Constant476/1 -> Product352/1
  Constant432/1 -> Product344/2
  Constant477/1 -> Product355/1
  Product338/1 -> Subtract253/2, Divide109/1
  Product346/1 -> Subtract267/2
  Constant470/1 -> Product349/1
  Subtract266/1 -> Divide102/2
  Constant451/1 -> Product342/2
  Subtract251/1 -> Product353/2
  Constant474/1 -> Subtract245/1
  Product342/1 -> Subtract257/1
  Product339/1 -> Subtract265/2
  Constant467/1 -> Product342/1
  Constant441/1 -> Subtract246/1
  Constant471/1 -> Product325/1
  Divide101/1 -> Product341/2
  Subtract269/1 -> Integrator72/1  "A'"
  Constant459/1 -> Subtract253/1
  Constant468/1 -> Product347/1
  Constant440/1 -> Math Function9/2
  Subtract265/1 -> Integrator76/1  "Sstemcells'"
  Product340/1 -> Subtract256/2, Divide101/1
  Constant449/1 -> Product327/1
  Constant455/1 -> Subtract244/1
  Constant442/1 -> Product326/1
  Subtract257/1 -> Integrator77/1  "Cyt'"
  Product350/1 -> Subtract261/1
  Subtract248/1 -> Divide106/1
  Divide102/1 -> Product350/1
  Product330/1 -> Divide107/1
  Product344/1 -> Product324/1
  Subtract250/1 -> Divide107/2
  Subtract249/1 -> Divide106/2
  Constant465/1 -> Subtract260/1
  Constant450/1 -> Product341/1
  Divide104/1 -> Subtract261/2
  Subtract262/1 -> Integrator75/1  "CLV3'"
  Constant478/1 -> Product354/1
  Constant433/1 -> Subtract266/1
  Constant454/1 -> Product332/1
  Product349/1 -> Subtract259/3
  Product326/1 -> Subtract249/3
  Product327/1 -> Subtract247/2
  Constant464/1 -> Product340/1
  Product348/1 -> Subtract258/3
  Subtract252/1 -> Divide108/2
  Product332/1 -> Subtract263/2
  Constant461/1 -> Subtract252/1
  Product335/1 -> Divide108/1, Subtract252/2
  Product358/1 -> Subtract269/2
  Product337/1 -> Product334/2
  Constant439/1 -> Product359/1
  Constant453/1 -> Product328/1
  Subtract258/1 -> Product354/2
  Subtract255/1 -> Product352/2
  Integrator73/1 -> Product327/2, Product340/2, Math Function9/1, i = 6/4  "6WUS"
  Constant445/1 -> Subtract249/1
  Constant457/1 -> Product334/1
  Product343/1 -> Subtract257/2
  Constant472/1 -> Subtract267/1, Divide103/1
  Subtract253/1 -> Divide109/2
  Constant446/1 -> Product338/1
  Subtract245/1 -> Divide105/1
  Integrator74/1 -> Product347/2, Product332/2, Subtract282/1, Product335/2, Subtract228/2, i = 6/5  "6CLV3signal"
  Constant435/1 -> Subtract264/1
  Product331/1 -> Subtract250/2
  Subtract244/1 -> Divide99/2
  Integrator78/1 -> Subtract260/2, Product325/2, Product336/1, Subtract243/2, i = 6/1  "6AHPTp"
  Subtract267/1 -> Divide103/2
  Constant436/1 -> Product356/1
  Constant448/1 -> Product329/1
  Constant437/1 -> Product358/1
  Constant463/1 -> Subtract256/1
  Product334/1 -> Subtract262/1
  Subtract260/1 -> Divide100/2
  Integrator75/1 -> Subtract278/1, Product333/2, Product345/2, Product326/2, Subtract224/2, i = 6/6  "6CLV3"
  Constant462/1 -> Product343/1
  Product324/1 -> Divide99/1
  Constant475/1 -> Product346/2
  Constant460/1 -> Product339/1
  Divide107/1 -> Product329/2
  Constant444/1 -> Subtract243/1
  Subtract246/1 -> Divide105/2
  Product351/1 -> Divide104/1
  Divide105/1 -> Subtract269/1
  Subtract268/1 -> Divide104/2
  Product329/1 -> Subtract263/1
  Product341/1 -> Subtract265/1
  Divide99/1 -> Subtract254/1
  Product357/1 -> Subtract246/3
  Subtract263/1 -> Integrator74/1  "CLV3signal'"
  Product325/1 -> Divide100/1
  Product359/1 -> Subtract249/2, Subtract248/2
  Integrator77/1 -> Subtract232/2, Product344/1, i = 6/8, Subtract286/1, Product349/2, Product343/2  "6Cyt"
  Integrator76/1 -> Product338/2, Product331/2, Product330/2, Subtract231/2, i = 6/7, Subtract285/1, Product348/2, Product339/2  "6Sstemcells"
  Subtract259/1 -> Product355/2
  Constant438/1 -> Product357/1
  Constant473/1 -> Product353/1
  Divide108/1 -> Product337/1
  Product352/1 -> Subtract263/3
  Divide109/1 -> Product337/2
  Subtract256/1 -> Divide101/2
  Divide106/1 -> Subtract247/1
  Constant469/1 -> Product348/1
  Constant458/1 -> Product333/1
  Product336/1 -> Divide102/1
  Constant466/1 -> Product345/1
  Constant479/1 -> Product351/1
  Constant443/1 -> Subtract248/1
  Constant452/1 -> Subtract250/1
  Constant447/1 -> Product328/2, Product331/1
  Product347/1 -> Subtract255/3
  Subtract261/1 -> Integrator79/1  "Bp'"
  Subtract291/1 -> Subtract293/2, Product372/2  "B"
  Product364/1 -> Product366/1
  Divide111/1 -> Subtract281/2
  Product389/1 -> Subtract289/3
  Product381/1 -> Subtract278/3
  Divide114/1 -> Product386/2
  Subtract274/1 -> Integrator81/1  "WUS'"
  Integrator80/1 -> Product394/2, Product382/1, i = 7/3  "7A"
  Constant504/1 -> Product371/1
  Subtract270/1 -> Subtract271/2, Product360/2  "AHPT"
  Integrator87/1 -> Subtract295/2, Product387/2, Subtract291/2, Product395/2, Product392/2, i = 7/2  "7Bp"
  Constant482/1 -> Subtract295/1
  Product390/1 -> Subtract292/3
  Math Function10/1 -> Product393/2
  Product391/1 -> Subtract284/3
  Subtract281/1 -> Integrator86/1  "AHPTp'"
  Product392/1 -> Subtract273/2, Subtract272/2
  Product369/1 -> Subtract289/2
  Constant524/1 -> Product388/1
  Constant480/1 -> Product380/2
  Constant525/1 -> Product391/1
  Product374/1 -> Subtract280/2, Divide120/1
  Product382/1 -> Subtract294/2
  Constant518/1 -> Product385/1
  Subtract293/1 -> Divide113/2
  Constant499/1 -> Product378/2
  Subtract278/1 -> Product389/2
  Constant522/1 -> Subtract272/1
  Product378/1 -> Subtract284/1
  Product375/1 -> Subtract292/2
  Constant515/1 -> Product378/1
  Constant489/1 -> Subtract273/1
  Constant519/1 -> Product361/1
  Divide112/1 -> Product377/2
  Subtract296/1 -> Integrator80/1  "A'"
  Constant507/1 -> Subtract280/1
  Constant516/1 -> Product383/1
  Constant488/1 -> Math Function10/2
  Subtract292/1 -> Integrator84/1  "Sstemcells'"
  Product376/1 -> Subtract283/2, Divide112/1
  Constant497/1 -> Product363/1
  Constant503/1 -> Subtract271/1
  Constant490/1 -> Product362/1
  Subtract284/1 -> Integrator85/1  "Cyt'"
  Product386/1 -> Subtract288/1
  Subtract275/1 -> Divide117/1
  Divide113/1 -> Product386/1
  Product366/1 -> Divide118/1
  Product380/1 -> Product360/1
  Subtract277/1 -> Divide118/2
  Subtract276/1 -> Divide117/2
  Constant513/1 -> Subtract287/1
  Constant498/1 -> Product377/1
  Divide115/1 -> Subtract288/2
  Subtract289/1 -> Integrator83/1  "CLV3'"
  Constant526/1 -> Product390/1
  Constant481/1 -> Subtract293/1
  Constant502/1 -> Product368/1
  Product385/1 -> Subtract286/3
  Product362/1 -> Subtract276/3
  Product363/1 -> Subtract274/2
  Constant512/1 -> Product376/1
  Product384/1 -> Subtract285/3
  Subtract279/1 -> Divide119/2
  Product368/1 -> Subtract290/2
  Constant509/1 -> Subtract279/1
  Product371/1 -> Divide119/1, Subtract279/2
  Product394/1 -> Subtract296/2
  Product373/1 -> Product370/2
  Constant487/1 -> Product395/1
  Constant501/1 -> Product364/1
  Subtract285/1 -> Product390/2
  Subtract282/1 -> Product388/2
  Integrator81/1 -> Product363/2, Product376/2, Math Function10/1, i = 7/4  "7WUS"
  Constant493/1 -> Subtract276/1
  Constant505/1 -> Product370/1
  Product379/1 -> Subtract284/2
  Constant520/1 -> Subtract294/1, Divide114/1
  Subtract280/1 -> Divide120/2
  Constant494/1 -> Product374/1
  Subtract272/1 -> Divide116/1
  Integrator82/1 -> Product383/2, Product368/2, Subtract309/1, Product371/2, Subtract255/2, i = 7/5  "7CLV3signal"
  Constant483/1 -> Subtract291/1
  Product367/1 -> Subtract277/2
  Subtract271/1 -> Divide110/2
  Integrator86/1 -> Subtract287/2, Product361/2, Product372/1, Subtract270/2, i = 7/1  "7AHPTp"
  Subtract294/1 -> Divide114/2
  Constant484/1 -> Product392/1
  Constant496/1 -> Product365/1
  Constant485/1 -> Product394/1
  Constant511/1 -> Subtract283/1
  Product370/1 -> Subtract289/1
  Subtract287/1 -> Divide111/2
  Integrator83/1 -> Subtract305/1, Product369/2, Product381/2, Product362/2, Subtract251/2, i = 7/6  "7CLV3"
  Constant510/1 -> Product379/1
  Product360/1 -> Divide110/1
  Constant523/1 -> Product382/2
  Constant508/1 -> Product375/1
  Divide118/1 -> Product365/2
  Constant492/1 -> Subtract270/1
  Subtract273/1 -> Divide116/2
  Product387/1 -> Divide115/1
  Divide116/1 -> Subtract296/1
  Subtract295/1 -> Divide115/2
  Product365/1 -> Subtract290/1
  Product377/1 -> Subtract292/1
  Divide110/1 -> Subtract281/1
  Product393/1 -> Subtract273/3
  Subtract290/1 -> Integrator82/1  "CLV3signal'"
  Product361/1 -> Divide111/1
  Product395/1 -> Subtract276/2, Subtract275/2
  Integrator85/1 -> Subtract259/2, Product380/1, i = 7/8, Subtract313/1, Product385/2, Product379/2  "7Cyt"
  Integrator84/1 -> Product374/2, Product367/2, Product366/2, Subtract258/2, i = 7/7, Subtract312/1, Product384/2, Product375/2  "7Sstemcells"
  Subtract286/1 -> Product391/2
  Constant486/1 -> Product393/1
  Constant521/1 -> Product389/1
  Divide119/1 -> Product373/1
  Product388/1 -> Subtract290/3
  Divide120/1 -> Product373/2
  Subtract283/1 -> Divide112/2
  Divide117/1 -> Subtract274/1
  Constant517/1 -> Product384/1
  Constant506/1 -> Product369/1
  Product372/1 -> Divide113/1
  Constant514/1 -> Product381/1
  Constant527/1 -> Product387/1
  Constant491/1 -> Subtract275/1
  Constant500/1 -> Subtract277/1
  Constant495/1 -> Product364/2, Product367/1
  Product383/1 -> Subtract282/3
  Subtract288/1 -> Integrator87/1  "Bp'"
  Subtract318/1 -> Subtract320/2, Product408/2  "B"
  Product400/1 -> Product402/1
  Divide122/1 -> Subtract308/2
  Product425/1 -> Subtract316/3
  Product417/1 -> Subtract305/3
  Divide125/1 -> Product422/2
  Subtract301/1 -> Integrator89/1  "WUS'"
  Integrator88/1 -> Product430/2, Product418/1, i = 8/3  "8A"
  Constant552/1 -> Product407/1
  Subtract297/1 -> Subtract298/2, Product396/2  "AHPT"
  Integrator95/1 -> Subtract322/2, Product423/2, Subtract318/2, Product431/2, Product428/2, i = 8/2  "8Bp"
  Constant530/1 -> Subtract322/1
  Product426/1 -> Subtract319/3
  Math Function11/1 -> Product429/2
  Product427/1 -> Subtract311/3
  Subtract308/1 -> Integrator94/1  "AHPTp'"
  Product428/1 -> Subtract300/2, Subtract299/2
  Product405/1 -> Subtract316/2
  Constant572/1 -> Product424/1
  Constant528/1 -> Product416/2
  Constant573/1 -> Product427/1
  Product410/1 -> Subtract307/2, Divide131/1
  Product418/1 -> Subtract321/2
  Constant566/1 -> Product421/1
  Subtract320/1 -> Divide124/2
  Constant547/1 -> Product414/2
  Subtract305/1 -> Product425/2
  Constant570/1 -> Subtract299/1
  Product414/1 -> Subtract311/1
  Product411/1 -> Subtract319/2
  Constant563/1 -> Product414/1
  Constant537/1 -> Subtract300/1
  Constant567/1 -> Product397/1
  Divide123/1 -> Product413/2
  Subtract323/1 -> Integrator88/1  "A'"
  Constant555/1 -> Subtract307/1
  Constant564/1 -> Product419/1
  Constant536/1 -> Math Function11/2
  Subtract319/1 -> Integrator92/1  "Sstemcells'"
  Product412/1 -> Subtract310/2, Divide123/1
  Constant545/1 -> Product399/1
  Constant551/1 -> Subtract298/1
  Constant538/1 -> Product398/1
  Subtract311/1 -> Integrator93/1  "Cyt'"
  Product422/1 -> Subtract315/1
  Subtract302/1 -> Divide128/1
  Divide124/1 -> Product422/1
  Product402/1 -> Divide129/1
  Product416/1 -> Product396/1
  Subtract304/1 -> Divide129/2
  Subtract303/1 -> Divide128/2
  Constant561/1 -> Subtract314/1
  Constant546/1 -> Product413/1
  Divide126/1 -> Subtract315/2
  Subtract316/1 -> Integrator91/1  "CLV3'"
  Constant574/1 -> Product426/1
  Constant529/1 -> Subtract320/1
  Constant550/1 -> Product404/1
  Product421/1 -> Subtract313/3
  Product398/1 -> Subtract303/3
  Product399/1 -> Subtract301/2
  Constant560/1 -> Product412/1
  Product420/1 -> Subtract312/3
  Subtract306/1 -> Divide130/2
  Product404/1 -> Subtract317/2
  Constant557/1 -> Subtract306/1
  Product407/1 -> Divide130/1, Subtract306/2
  Product430/1 -> Subtract323/2
  Product409/1 -> Product406/2
  Constant535/1 -> Product431/1
  Constant549/1 -> Product400/1
  Subtract312/1 -> Product426/2
  Subtract309/1 -> Product424/2
  Integrator89/1 -> Product399/2, Product412/2, Math Function11/1, i = 8/4  "8WUS"
  Constant541/1 -> Subtract303/1
  Constant553/1 -> Product406/1
  Product415/1 -> Subtract311/2
  Constant568/1 -> Subtract321/1, Divide125/1
  Subtract307/1 -> Divide131/2
  Constant542/1 -> Product410/1
  Subtract299/1 -> Divide127/1
  Integrator90/1 -> Product419/2, Product404/2, Product407/2, Subtract282/2, i = 8/5  "8CLV3signal"
  Constant531/1 -> Subtract318/1
  Product403/1 -> Subtract304/2
  Subtract298/1 -> Divide121/2
  Integrator94/1 -> Subtract314/2, Product397/2, Product408/1, Subtract297/2, i = 8/1  "8AHPTp"
  Subtract321/1 -> Divide125/2
  Constant532/1 -> Product428/1
  Constant544/1 -> Product401/1
  Constant533/1 -> Product430/1
  Constant559/1 -> Subtract310/1
  Product406/1 -> Subtract316/1
  Subtract314/1 -> Divide122/2
  Integrator91/1 -> Product405/2, Product417/2, Product398/2, Subtract278/2, i = 8/6  "8CLV3"
  Constant558/1 -> Product415/1
  Product396/1 -> Divide121/1
  Constant571/1 -> Product418/2
  Constant556/1 -> Product411/1
  Divide129/1 -> Product401/2
  Constant540/1 -> Subtract297/1
  Subtract300/1 -> Divide127/2
  Product423/1 -> Divide126/1
  Divide127/1 -> Subtract323/1
  Subtract322/1 -> Divide126/2
  Product401/1 -> Subtract317/1
  Product413/1 -> Subtract319/1
  Divide121/1 -> Subtract308/1
  Product429/1 -> Subtract300/3
  Subtract317/1 -> Integrator90/1  "CLV3signal'"
  Product397/1 -> Divide122/1
  Product431/1 -> Subtract303/2, Subtract302/2
  Integrator93/1 -> Subtract286/2, Product416/1, i = 8/8, Product421/2, Product415/2  "8Cyt"
  Integrator92/1 -> Product410/2, Product403/2, Product402/2, Subtract285/2, i = 8/7, Product420/2, Product411/2  "8Sstemcells"
  Subtract313/1 -> Product427/2
  Constant534/1 -> Product429/1
  Constant569/1 -> Product425/1
  Divide130/1 -> Product409/1
  Product424/1 -> Subtract317/3
  Divide131/1 -> Product409/2
  Subtract310/1 -> Divide123/2
  Divide128/1 -> Subtract301/1
  Constant565/1 -> Product420/1
  Constant554/1 -> Product405/1
  Product408/1 -> Divide124/1
  Constant562/1 -> Product417/1
  Constant575/1 -> Product423/1
  Constant539/1 -> Subtract302/1
  Constant548/1 -> Subtract304/1
  Constant543/1 -> Product400/2, Product403/1
  Product419/1 -> Subtract309/3
  Subtract315/1 -> Integrator95/1  "Bp'"
